simulink model "model"  (R2024b)
settings: Solver=ode45  StartTime=0.0  StopTime=1  FixedStep=0.0000001  MaxStep=1e-5  RelTol=1e-9  AbsTol=1e-9
InitFcn:
  | rs=0.435
  | Lls=0.754/(2*pi*60)
  | rr=0.816
  | Llr=0.754/(2*pi*60)
  | Lm=26.13/(2*pi*60)
  | J=0.0089; % 0.089
  | p=4;
  | Lss=Lls+Lm;
  | Lrr=Llr+Lm;
  | n= 1710; %rpm
  | Freq = 60;
  | 
  | Pbase= 3*746; % kw, 3hp
  | Vbase=220/sqrt(3)
  | Ibase= 8.2
  | Zbase = Vbase/Ibase
  | Lbase=Zbase/(2*pi*60)
  | Lm_pu = Lm/Lbase
  | Flx_pu = 1/Lm_pu
  | We_rated = 2*pi*Freq
  | Wm_rated = n/60*2*pi
  | T_rated = Pbase/Wm_rated
  | Flux_base = Vbase*sqrt(2)/We_rated
libraries: powerlib_extras x6, simulink_extras x1, spspowerguiLib x1
settings Model: Creator=Aditya  LastModifiedBy=tnt4
settings SolverCC: AutoScaleAbsTol=off  ZeroCrossAlgorithm=Adaptive  AlgebraicLoopSolver=TrustRegion
settings DataIOCC: SaveFormat=Array  SignalLoggingSaveFormat=ModelDataLogs  ReturnWorkspaceOutputs=off
settings OptimizationCC: BlockReduction=off  BooleanDataType=off  ExpressionDepthLimit=2147483647  InitFltsAndDblsToZero=on  LifeSpan=inf
settings DebuggingCC: SaveWithParameterizedLinksMsg=none  UnderspecifiedInitializationDetection=Classic  MergeDetectMultiDrivingBlocksExec=none  SignalResolutionControl=TryResolveAllWithWarning  MaxConsecutiveZCsMsg=none  MultiTaskDSMMsg=warning  MultiTaskCondExecSysMsg=none  FcnCallInpInsideContextMsg=warning  UnconnectedInputMsg=warning  UnconnectedOutputMsg=warning  UnconnectedLineMsg=warning  StateNameClashWarn=warning  SFUnexpectedBacktrackingDiag=warning  SFNoUnconditionalDefaultTransitionDiag=warning  SFExecutionAtInitializationDiag=none  ArithmeticOperatorsInVariantConditions=warning
settings HardwareCC: ProdBitPerPointer=32  ProdBitPerSizeT=32  ProdBitPerPtrDiffT=32  ProdLargestAtomicFloat=None  ProdIntDivRoundTo=Undefined  ProdEndianess=Unspecified  ProdWordSize=32  ProdHWDeviceType=32-bit Generic  TargetUnknown=on
settings ModelReferenceCC: EnableRefExpFcnMdlSchedulingChecks=on  PropagateSignalLabelsOutOfModel=off
settings SFSimCC: SimUseLocalCustomCode=off  CustomCodeUndefinedFunction=UseInterfaceOnly
settings RTWCC: TemplateMakefile=grt_unix.tmf  RTWUseLocalCustomCode=off  GPUComputeCapability=3.5
settings CodeAppCC: StateflowObjectComments=on
settings GRTTargetCC: TargetFcnLib=ansi_tfl_tmw.mat  TargetLangStandard=C89/C90 (ANSI)  CombineOutputUpdateFcns=off  GRTInterface=on
settings ConfigComp: CovMetricSettings=dw  CovSaveCumulativeToWorkspaceVar=on  CovSaveSingleToWorkspaceVar=on  CovExternalEMLEnable=off

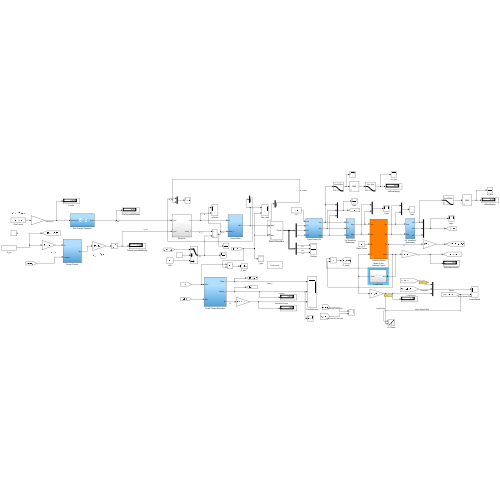
[thumbnail: Simulink's stored preview of the top-level diagram]
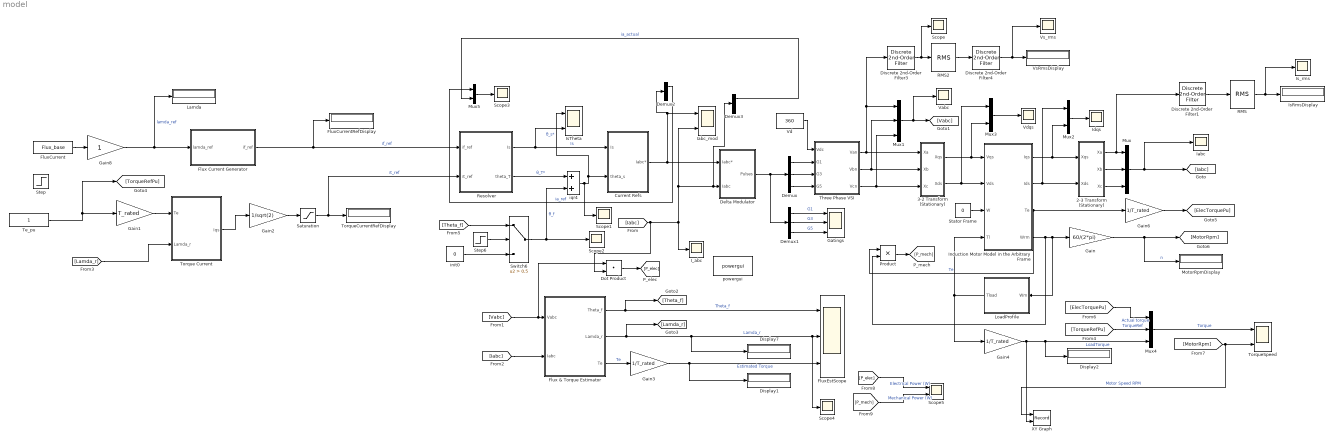
== system model ==
  2-3 Transform (Stationary) : Subsystem
  3-2 Transform (Stationary) : Subsystem
  Current Refs : Subsystem
  Delta Modulator : Subsystem  AncestorBlock=electricdrivelib/Fundamental Drive Blocks/Field-Oriented Controller/Detailed/Current Regulator  mask{h=Ibase*0.05}
      mask prompts: h "Modulator Band Width"
  Demux{,1..3} (4 alike) : Demux  Outputs=3
  Discrete 2nd-Order Filter1 : powerlib_extras/Discrete  Control Blocks/Discrete  2nd-Order Filter  FilterType=Lowpass  Fo=300  Zeta=0.5  Ts=50e-6  Initialize=off  Vac_Init=[0.8 -25 60]  Vdc_Init=-0.4  PlotResponse=off  param1=[1 500 1]
  Discrete 2nd-Order Filter3 : powerlib_extras/Discrete  Control Blocks/Discrete  2nd-Order Filter  FilterType=Lowpass  Fo=300  Zeta=0.5  Ts=50e-6  Initialize=off  Vac_Init=[0.8 -25 60]  Vdc_Init=-0.4  PlotResponse=off  param1=[1 500 1]
  Discrete 2nd-Order Filter4 : powerlib_extras/Discrete  Control Blocks/Discrete  2nd-Order Filter  FilterType=Lowpass  Fo=1  Zeta=0.5  Ts=50e-6  Initialize=off  Vac_Init=[0.8 -25 60]  Vdc_Init=-0.4  PlotResponse=off  param1=[1 500 1]
  Display1 : Display
  Display2 : Display
  Display7 : Display
  Dot Product : DotProduct  OutDataTypeStr=Inherit: Inherit via internal rule
  Flux & Torque Estimator : Subsystem
  Flux Current Generator : Subsystem
  FluxCurrent : Constant  Value=Flux_base
  FluxCurrentRefDisplay : Display
  FluxEstScope : Scope  NumInputPorts=3
  Gain : Gain  Gain=60/(2*pi)
  Gain1 : Gain  Gain=T_rated
  Gain2 : Gain  Gain=1/sqrt(2)
  Gain3 : Gain  Gain=1/T_rated
  Gain4 : Gain  Gain=1/T_rated
  Gain6 : Gain  Gain=1/T_rated
  Gain8 : Gain
  Gatings : Scope  NumInputPorts=3
  I_abc : Scope
  Iabc : Scope
  Iabc_mod : Scope  NumInputPorts=2
  Idqs : Scope
  Induction Motor Model in the Arbitrary Frame : Subsystem  mask{Rs=rs, Rr=rr, XLm=Lm, XLs=Lls, XLr=Llr, J=J}
  IsRmsDisplay : Display
  IsTheta : Scope  NumInputPorts=2
  Is_rms : Scope
  Lamda : Display
  LoadProfile : Subsystem
  MotorRpmDisplay : Display
  Mux : Mux  Inputs=3
  Mux1 : Mux  Inputs=3
  Mux2 : Mux  Inputs=2
  Mux3 : Mux  Inputs=2
  Mux4 : Mux  Inputs=3
  Mux5 : Mux  Inputs=2
  Product : Product
  RMS : powerlib_extras/Measurements/RMS  f1=60
  RMS2 : powerlib_extras/Measurements/RMS  f1=60
  Resolver : Subsystem
  Saturation : Saturate  UpperLimit=Ibase*1.5  LowerLimit=-Ibase*1.5
  Scope{,1..4} (5 alike) : Scope
  Scope5 : Scope  NumInputPorts=2
  Stator Frame : Constant  Value=0
  Step : Step  Time=0.5  Before=0.2  SampleTime=0
  Step6 : Step  Time=0.01  SampleTime=0
  Switch6 : Switch  Criteria=u2 > Threshold  Threshold=0.5  SaturateOnIntegerOverflow=off  InputSameDT=off
  Te_pu : Constant
  Three Phase VSI : Subsystem
  "Torque Current " : Subsystem
  TorqueCurrentRefDisplay : Display
  TorqueSpeed : Scope  NumInputPorts=2
  Vabc : Scope
  Vd : Constant  Value=360
  Vdqs : Scope
  VsRmsDisplay : Display
  Vs_rms : Scope
  XY Graph : Record  FileSettingsInternal="{\"entries\":[{\"content\":{\"excelSettings\":{\"content\":{},\"type\":\"Streamout.ExcelSettings\"}},\"type\":\"Streamout.FileSettingStorage\",\"uuid\":\"\"}],\"packageUris\":[\"http:\\/\\/schema.mathworks.com\\/mf0\\/streamout_blocks\\/R2020a\"],\"version\":\"1.0\"}"  Layout=[1 1]  SignalsInternal="{\"entries\":[{\"content\":{\"signals\":[{\"content\":{\"blockPath\":[],\"dimensions\":[1],\"domain\":\"\",\"lineColor\":\"#a2142f\",\"plots\":[ 1 ],\"port\":1,\"sid\":[\"\"],\"signalID\":1,\"signalName\":\"Motor Speed RPM\"},\"type\":\"RecordBlkView.Signal\",\"uuid\":\"\"},{\"content\":{\"blockPath\":[],\"dimensions\":[1],\"domain\":\"\",\"lineColor\":\"#139fff\",\"plots\":[ 1 ],\"port\":2,\"sid\":[\"\"],\"signalID\":2,\"signalName\":\"LoadTorque\"},\"type\":\"RecordBlkView.Signal\",\"uuid\":\"\"}]},\"type\":\"RecordBlkView.InputSignals\",\"uuid\":\"\"}],\"packageUris\":[\"http:\\/\\/schema.mathworks.com\\/mf0\\/streamout_blocks\\/R2020a\"],\"version\":\"1.0\"}"  VisualizationBindings="{\"xyplotplugin\":{\"info\":[{\"series\":[{\"bindingParametersList\":[{\"parameter\":\"X-Axis\",\"signalID\":1,\"signalName\":\"Motor Speed RPM\"},{\"parameter\":\"Y-Axis\",\"signalID\":2,\"signalName\":\"LoadTorque\"}],\"seriesID\":0}],\"subplotID\":1}]}}"  CompatibilityTag=XY
  init0 : Constant  Value=0
  iqr4 : Sum
  powergui : spspowerguiLib/powergui  Priority=1  SimulationMode=Continuous  SampleTime=50e-6  frequency=60  Iterations=50  frequencyindice=60  Pbase=100e6  ErrMax=1e-4  UnitsV=kV  UnitsW=MW  buscounter=0  FunctionMessages=off  echomessages=off  EnableUseOfTLC=off  CurrentSourceSwitches=off  DisableSnubberDevices=off  DisableRonSwitches=off  DisableVfSwitches=off  DisplayEquations=off  AutomaticDiscreteSolvers=off  SolverType=Tustin/Backward Euler (TBE)  Interpol=off  ExternalGateDelay=off  methode=off  Ts=100  x0status=blocks  SPID=on  SwTol=0  HookPort=off  NonlinearTolerance=1e-4  nMaxIteration=100  ContinueOnMaxIteration=off  RestoreLinks=warning  ResistiveCurrentMeasurement=off  Frange=[0:2:500]  Ylog=off  Xlog=on  ShowGrid=off  save=off  variable=ZData  structure=0  ZoomFFT=off  StartTime=0.0  cycles=1  DisplayStyle=1  fundamental=60  FreqAxis=off  MaxFrequency=1000  frequencyindicesteady=1  RmsSteady=1  display=off
  wires:
  3-2 Transform (Stationary)/1(Xqs) -> Mux3/2, Induction Motor Model in the Arbitrary Frame/1(Vqs)
  3-2 Transform (Stationary)/2(Xds) -> Mux3/1, Induction Motor Model in the Arbitrary Frame/2(Vds)
  Stator Frame/1 -> Induction Motor Model in the Arbitrary Frame/3(W)
  Induction Motor Model in the Arbitrary Frame/1(Iqs) -> Mux2/2, 2-3 Transform (Stationary)/1(Xqs)
  Induction Motor Model in the Arbitrary Frame/2(Ids) -> Mux2/1, 2-3 Transform (Stationary)/2(Xds)
  Induction Motor Model in the Arbitrary Frame/4(Wrm) -> Product/2, LoadProfile/1(Wm), Gain/1
  Gain/1 -> [MotorRpm], MotorRpmDisplay/1  "n"
  Vd/1 -> Three Phase VSI/1(Vdc)
  Demux/1 -> Three Phase VSI/2(G1)
  Demux/2 -> Three Phase VSI/3(G3)
  Demux/3 -> Three Phase VSI/4(G5)
  2-3 Transform (Stationary)/2(Xb) -> Mux/2
  2-3 Transform (Stationary)/3(Xc) -> Mux/3
  2-3 Transform (Stationary)/1(Xa) -> Discrete 2nd-Order Filter1/1, Mux/1
  Three Phase VSI/1(Van) -> Discrete 2nd-Order Filter3/1, Mux1/1, 3-2 Transform (Stationary)/1(Xa)
  Three Phase VSI/2(Vbn) -> Mux1/2, 3-2 Transform (Stationary)/2(Xb)
  Three Phase VSI/3(Vcn) -> Mux1/3, 3-2 Transform (Stationary)/3(Xc)
  Mux1/1 -> Vabc/1, [Vabc]
  [Iabc] -> Dot Product/2, I_abc/1, Iabc_mod/2, Demux3/1, Delta Modulator/2(Iabc)
  Current Refs/1(Iabc*) -> Demux2/1, Iabc_mod/1, Delta Modulator/1(Iabc*)
  [Vabc] -> Dot Product/1, Flux & Torque Estimator/1(Vabc)
  [Iabc] -> Flux & Torque Estimator/2(Iabc)
  Flux & Torque Estimator/1(Theta_f) -> [Theta_f], FluxEstScope/1  "Theta_f"
  Flux & Torque Estimator/3(Te) -> Gain3/1  "Te"
  Induction Motor Model in the Arbitrary Frame/3(Te) -> Product/1, Gain6/1  "Te"
  Mux/1 -> [Iabc], Iabc/1
  Flux & Torque Estimator/2(Lamda_r) -> [Lamda_r], Display7/1, Scope4/1, FluxEstScope/2  "Lamda_r"
  FluxCurrent/1 -> Gain8/1
  iqr4/1 -> Scope1/1, IsTheta/1, Current Refs/2(theta_s)  "θ_s*"
  Delta Modulator/1(Pulses) -> Demux1/1, Demux/1
  Demux1/3 -> Gatings/3  "G5"
  Demux1/2 -> Gatings/2  "G3"
  Demux1/1 -> Gatings/1  "G1"
  Mux2/1 -> Idqs/1
  Mux3/1 -> Vdqs/1
  LoadProfile/1(Tload) -> Gain4/1, Induction Motor Model in the Arbitrary Frame/4(Tl)
  Gain3/1 -> Display1/1, FluxEstScope/3  "Estimated Torque"
  Discrete 2nd-Order Filter1/1 -> RMS/1
  RMS/1 -> Is_rms/1, IsRmsDisplay/1
  "Torque Current "/1(Iqs) -> Gain2/1
  Gain1/1 -> "Torque Current "/1(Te)
  Gain2/1 -> Saturation/1
  [Lamda_r] -> "Torque Current "/2(Lamda_r)
  Saturation/1 -> Resolver/2(it_ref), TorqueCurrentRefDisplay/1  "it_ref"
  RMS2/1 -> Discrete 2nd-Order Filter4/1
  Discrete 2nd-Order Filter3/1 -> Scope/1, RMS2/1
  Discrete 2nd-Order Filter4/1 -> Vs_rms/1, VsRmsDisplay/1
  Gain4/1 -> XY Graph/2, Display2/1, Mux4/3  "LoadTorque"
  [TorqueRefPu] -> Mux4/2  "TorqueRef"
  Gain6/1 -> [ElecTorquePu]
  [ElecTorquePu] -> Mux4/1  "Actual torque"
  Mux4/1 -> TorqueSpeed/1  "Torque"
  [MotorRpm] -> XY Graph/1, TorqueSpeed/2  "Motor Speed RPM"
  Gain8/1 -> Lamda/1, Flux Current Generator/1(lamda_ref)  "lamda_ref"
  [Theta_f] -> Switch6/1
  Step6/1 -> Switch6/2
  init0/1 -> Switch6/3
  Resolver/1(Is) -> IsTheta/2, Current Refs/1(Is)  "Is"
  Resolver/2(theta_T) -> iqr4/1  "θ_T*"
  Flux Current Generator/1(if_ref) -> FluxCurrentRefDisplay/1, Resolver/1(if_ref)  "if_ref"
  Switch6/1 -> iqr4/2, Scope2/1  "θ_f"
  Mux5/1 -> Scope3/1
  Demux2/1 -> Mux5/1  "ia_ref"
  Demux3/1 -> Mux5/2  "ia_actual"
  Te_pu/1 -> Gain1/1, [TorqueRefPu]
  Dot Product/1 -> [P_elec]
  Product/1 -> [P_mech]
  [P_elec] -> Scope5/1  "Electrical Power (W)"
  [P_mech] -> Scope5/2  "Mechanical Power (W)"

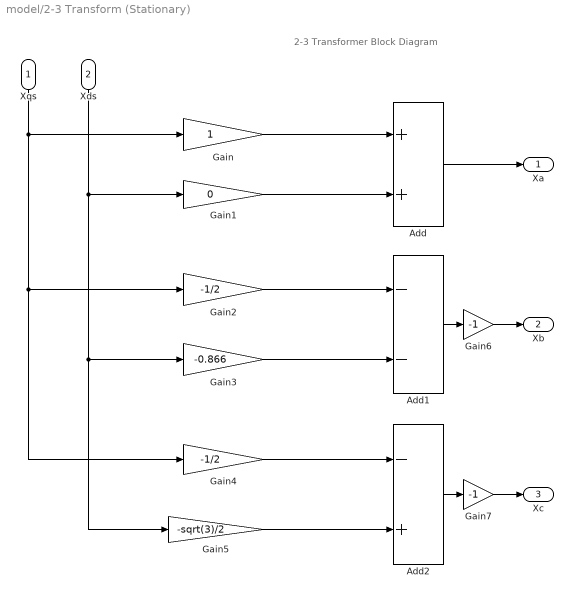
== system model/2-3 Transform (Stationary) ==
  note: 2-3 Transformer Block Diagram
  Xqs : Inport
  Xds : Inport  Port=2
  Add : Sum
  Add1 : Sum  Inputs=--
  Add2 : Sum  Inputs=-+
  Gain : Gain
  Gain1 : Gain  Gain=0
  Gain2 : Gain  Gain=-1/2
  Gain3 : Gain  Gain=-0.866
  Gain4 : Gain  Gain=-1/2
  Gain5 : Gain  Gain=-sqrt(3)/2
  Gain6 : Gain  Gain=-1
  Gain7 : Gain  Gain=-1
  Xa : Outport  VectorParamsAs1DForOutWhenUnconnected=off
  Xb : Outport  Port=2  VectorParamsAs1DForOutWhenUnconnected=off
  Xc : Outport  Port=3  VectorParamsAs1DForOutWhenUnconnected=off
  wires:
  Add2/1 -> Gain7/1
  Gain/1 -> Add/1
  Gain3/1 -> Add1/2
  Gain5/1 -> Add2/2
  Gain1/1 -> Add/2
  Gain7/1 -> Xc/1
  Xds/1 -> Gain1/1, Gain3/1, Gain5/1
  Add1/1 -> Gain6/1
  Gain2/1 -> Add1/1
  Xqs/1 -> Gain/1, Gain2/1, Gain4/1
  Gain6/1 -> Xb/1
  Gain4/1 -> Add2/1
  Add/1 -> Xa/1

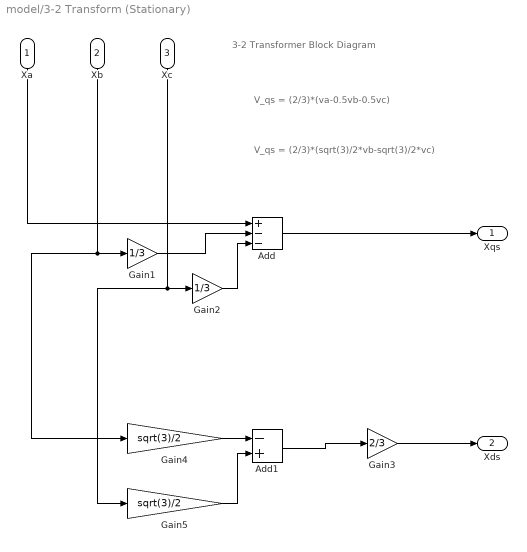
== system model/3-2 Transform (Stationary) ==
  note: 3-2 Transformer Block Diagram
  note: V_qs = (2/3)*(sqrt(3)/2*vb-sqrt(3)/2*vc)
  note: V_qs = (2/3)*(va-0.5vb-0.5vc)
  Xa : Inport
  Xb : Inport  Port=2
  Xc : Inport  Port=3
  Add : Sum  Inputs=+--
  Add1 : Sum  Inputs=-+
  Gain1 : Gain  Gain=1/3
  Gain2 : Gain  Gain=1/3
  Gain3 : Gain  Gain=2/3
  Gain4 : Gain  Gain=sqrt(3)/2
  Gain5 : Gain  Gain=sqrt(3)/2
  Xqs : Outport  VectorParamsAs1DForOutWhenUnconnected=off
  Xds : Outport  Port=2  VectorParamsAs1DForOutWhenUnconnected=off
  wires:
  Gain5/1 -> Add1/2
  Add/1 -> Xqs/1
  Add1/1 -> Gain3/1
  Gain1/1 -> Add/2
  Gain2/1 -> Add/3
  Xa/1 -> Add/1
  Xc/1 -> Gain5/1, Gain2/1
  Xb/1 -> Gain4/1, Gain1/1
  Gain4/1 -> Add1/1
  Gain3/1 -> Xds/1

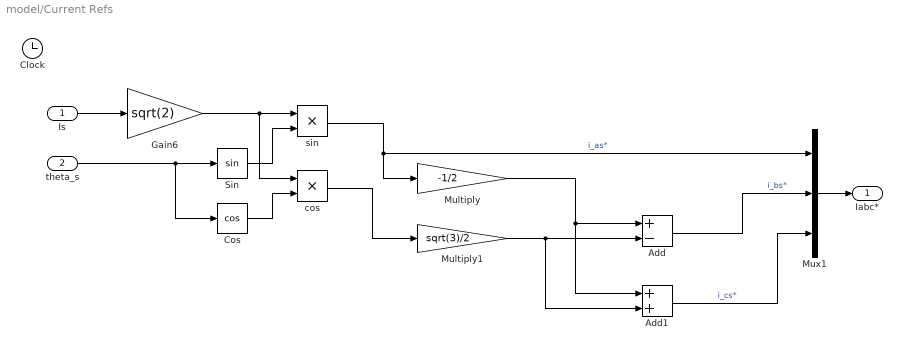
== system model/Current Refs ==
  Is : Inport
  theta_s : Inport  Port=2
  Add : Sum  Inputs=+-
  Add1 : Sum
  Clock : Clock
  Cos : Trigonometry  Operator=cos
  Gain6 : Gain  Gain=sqrt(2)
  Multiply : Gain  Gain=-1/2
  Multiply1 : Gain  Gain=sqrt(3)/2
  Mux1 : Mux  Inputs=3
  Sin : Trigonometry
  cos : Product
  sin : Product
  Iabc* : Outport  VectorParamsAs1DForOutWhenUnconnected=off
  wires:
  Mux1/1 -> Iabc*/1
  Is/1 -> Gain6/1
  cos/1 -> Multiply1/1
  sin/1 -> Mux1/1, Multiply/1  "i_as*"
  Add/1 -> Mux1/2  "i_bs*"
  Multiply1/1 -> Add1/2, Add/2
  Multiply/1 -> Add1/1, Add/1
  Add1/1 -> Mux1/3  "i_cs*"
  Sin/1 -> sin/2
  Cos/1 -> cos/2
  Gain6/1 -> cos/1, sin/1
  theta_s/1 -> Cos/1, Sin/1

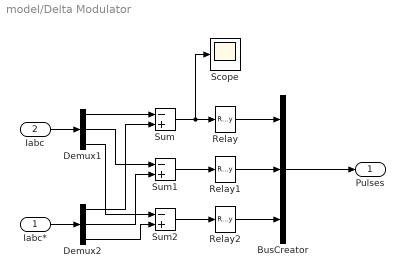
== system model/Delta Modulator ==
  Iabc* : Inport
  Iabc : Inport  Port=2
  BusCreator : BusCreator  Inputs=3
  Demux1 : Demux  Outputs=3
      settings: DisplayOption=none
  Demux2 : Demux  Outputs=3
      settings: DisplayOption=none
  Relay : Relay  OnSwitchValue=1/2  OffSwitchValue=-1/2
  Relay1 : Relay  OnSwitchValue=1/2  OffSwitchValue=-1/2
  Relay2 : Relay  OnSwitchValue=1/2  OffSwitchValue=-1/2
  Scope : Scope
  Sum : Sum  Inputs=-+  InputSameDT=on  SaturateOnIntegerOverflow=on  OutDataTypeStr=Inherit: Same as first input
  Sum1 : Sum  Inputs=-+  InputSameDT=on  SaturateOnIntegerOverflow=on  OutDataTypeStr=Inherit: Same as first input
  Sum2 : Sum  Inputs=-+  InputSameDT=on  SaturateOnIntegerOverflow=on  OutDataTypeStr=Inherit: Same as first input
  Pulses : Outport  InitialOutput=0  VectorParamsAs1DForOutWhenUnconnected=off
  wires:
  Sum/1 -> Scope/1, Relay/1
  Sum1/1 -> Relay1/1
  Demux1/1 -> Sum/1
  Demux1/2 -> Sum1/1
  BusCreator/1 -> Pulses/1
  Iabc/1 -> Demux1/1
  Sum2/1 -> Relay2/1
  Demux1/3 -> Sum2/1
  Demux2/3 -> Sum2/2
  Demux2/2 -> Sum1/2
  Demux2/1 -> Sum/2
  Iabc*/1 -> Demux2/1
  Relay/1 -> BusCreator/1
  Relay1/1 -> BusCreator/2
  Relay2/1 -> BusCreator/3

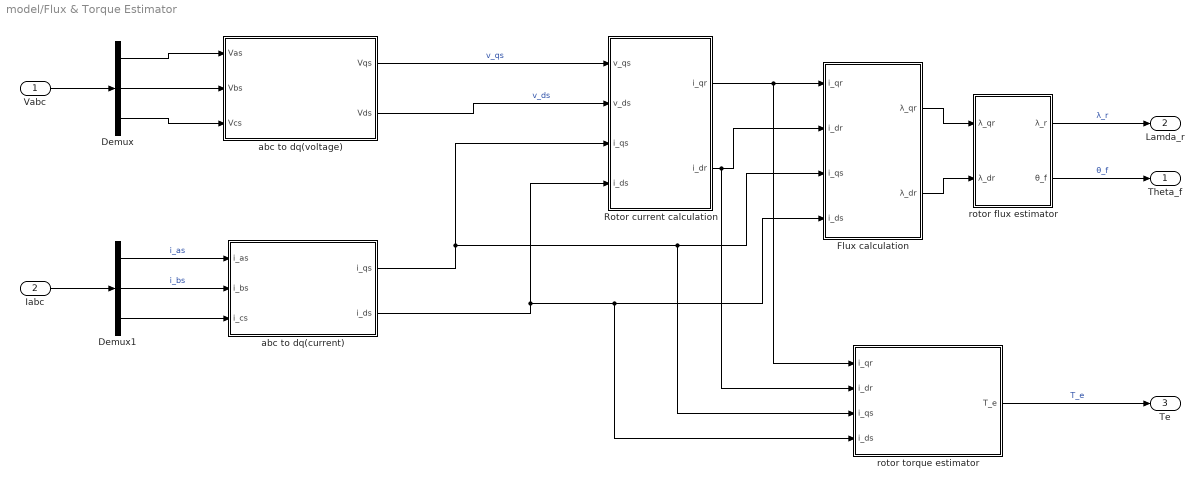
== system model/Flux & Torque Estimator ==
  Vabc : Inport
  Iabc : Inport  Port=2
  Demux : Demux  Outputs=3
  Demux1 : Demux  Outputs=3
  Flux calculation : Subsystem
  Rotor current calculation : Subsystem
  abc to dq(current) : Subsystem
  abc to dq(voltage) : Subsystem
  rotor flux estimator : Subsystem
  rotor torque estimator : Subsystem
  Theta_f : Outport  OutDataTypeStr=double  VectorParamsAs1DForOutWhenUnconnected=off
  Lamda_r : Outport  Port=2  VectorParamsAs1DForOutWhenUnconnected=off
  Te : Outport  Port=3  VectorParamsAs1DForOutWhenUnconnected=off
  wires:
  Vabc/1 -> Demux/1
  Iabc/1 -> Demux1/1
  abc to dq(current)/2(i_ds) -> rotor torque estimator/4(i_ds), Flux calculation/4(i_ds), Rotor current calculation/4(i_ds)
  abc to dq(voltage)/1(Vqs) -> Rotor current calculation/1(v_qs)  "v_qs"
  Rotor current calculation/1(i_qr) -> rotor torque estimator/1(i_qr), Flux calculation/1(i_qr)
  Flux calculation/2(λ_dr) -> rotor flux estimator/2(λ_dr)
  Demux/2 -> abc to dq(voltage)/2(Vbs)
  rotor flux estimator/2(θ_f) -> Theta_f/1  "θ_f"
  Rotor current calculation/2(i_dr) -> rotor torque estimator/2(i_dr), Flux calculation/2(i_dr)
  rotor torque estimator/1(T_e) -> Te/1  "T_e"
  rotor flux estimator/1(λ_r) -> Lamda_r/1  "λ_r"
  abc to dq(current)/1(i_qs) -> Rotor current calculation/3(i_qs), rotor torque estimator/3(i_qs), Flux calculation/3(i_qs)
  abc to dq(voltage)/2(Vds) -> Rotor current calculation/2(v_ds)  "v_ds"
  Flux calculation/1(λ_qr) -> rotor flux estimator/1(λ_qr)
  Demux1/1 -> abc to dq(current)/1(i_as)  "i_as"
  Demux/1 -> abc to dq(voltage)/1(Vas)
  Demux/3 -> abc to dq(voltage)/3(Vcs)
  Demux1/2 -> abc to dq(current)/2(i_bs)  "i_bs"
  Demux1/3 -> abc to dq(current)/3(i_cs)

== system model/Flux Current Generator ==
  lamda_ref : Inport
  Gain7 : Gain  Gain=1/Lm
  Gain9 : Gain  Gain=1/sqrt(2)
  if_ref : Outport
  wires:
  Gain7/1 -> Gain9/1
  Gain9/1 -> if_ref/1  "if_ref"
  lamda_ref/1 -> Gain7/1

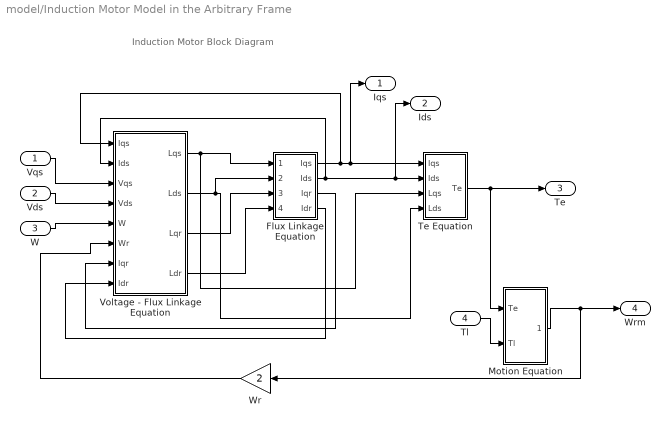
== system model/Induction Motor Model in the Arbitrary Frame ==
  note: Induction Motor Block Diagram
  Vqs : Inport
  Vds : Inport  Port=2
  W : Inport  Port=3
  Tl : Inport  Port=4
  Flux Linkage Equation : Subsystem
  Motion Equation : Subsystem
  Te Equation : Subsystem
  Voltage - Flux Linkage Equation : Subsystem
  Wr : Gain  Gain=2
  Iqs : Outport  VectorParamsAs1DForOutWhenUnconnected=off
  Ids : Outport  Port=2  VectorParamsAs1DForOutWhenUnconnected=off
  Te : Outport  Port=3  VectorParamsAs1DForOutWhenUnconnected=off
  Wrm : Outport  Port=4  VectorParamsAs1DForOutWhenUnconnected=off
  wires:
  Flux Linkage Equation/1(Iqs) -> Voltage - Flux Linkage Equation/1(Iqs), Te Equation/1(Iqs), Iqs/1
  Flux Linkage Equation/2(Ids) -> Voltage - Flux Linkage Equation/2(Ids), Te Equation/2(Ids), Ids/1
  Te Equation/1(Te) -> Motion Equation/1(Te), Te/1
  Motion Equation/1(Wrm) -> Wr/1, Wrm/1
  Wr/1 -> Voltage - Flux Linkage Equation/6(Wr)
  Flux Linkage Equation/3(Iqr) -> Voltage - Flux Linkage Equation/7(Iqr)
  Flux Linkage Equation/4(Idr) -> Voltage - Flux Linkage Equation/8(Idr)
  Vqs/1 -> Voltage - Flux Linkage Equation/3(Vqs)
  Vds/1 -> Voltage - Flux Linkage Equation/4(Vds)
  W/1 -> Voltage - Flux Linkage Equation/5(W)
  Tl/1 -> Motion Equation/2(Tl)
  Voltage - Flux Linkage Equation/1(Lqs) -> Flux Linkage Equation/1(Lqs), Te Equation/3(Lqs)
  Voltage - Flux Linkage Equation/2(Lds) -> Flux Linkage Equation/2(Lds), Te Equation/4(Lds)
  Voltage - Flux Linkage Equation/3(Lqr) -> Flux Linkage Equation/3(Lqr)
  Voltage - Flux Linkage Equation/4(Ldr) -> Flux Linkage Equation/4(Ldr)

== system model/LoadProfile ==
  Wm : Inport
  Add : Sum
  FanTypeTrqGain : Constant  Value=T_rated/(Wm_rated^2)
  Multiply1 : Product  Inputs=3
  Step : Step  Time=0.5  After=0  SampleTime=0
  Tload : Outport  VectorParamsAs1DForOutWhenUnconnected=off
  wires:
  Wm/1 -> Multiply1/2, Multiply1/1
  FanTypeTrqGain/1 -> Multiply1/3
  Multiply1/1 -> Add/1
  Step/1 -> Add/2
  Add/1 -> Tload/1

== system model/Resolver ==
  if_ref : Inport
  it_ref : Inport  Port=2
  Cartesian to Polar : simulink_extras/Transformations/Cartesian to Polar
  Is : Outport
  theta_T : Outport  Port=2
  wires:
  Cartesian to Polar/2 -> theta_T/1  "theta_T"
  Cartesian to Polar/1 -> Is/1  "Is"
  it_ref/1 -> Cartesian to Polar/2
  if_ref/1 -> Cartesian to Polar/1

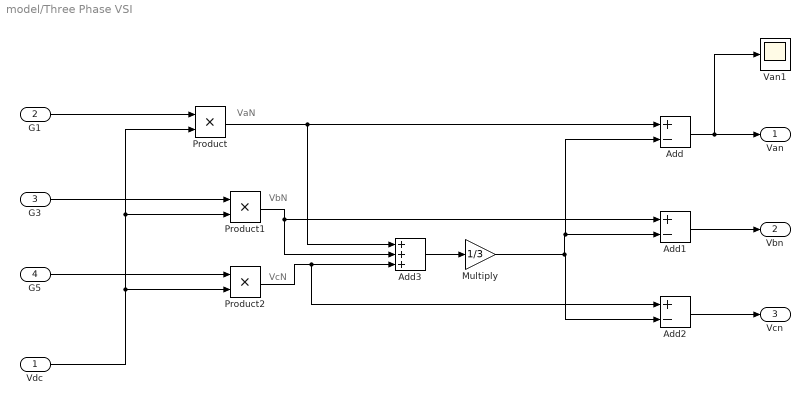
== system model/Three Phase VSI ==
  note: VaN
  note: VbN
  note: VcN
  Vdc : Inport
  G1 : Inport  Port=2
  G3 : Inport  Port=3
  G5 : Inport  Port=4
  Add : Sum  Inputs=+-
  Add1 : Sum  Inputs=+-
  Add2 : Sum  Inputs=+-
  Add3 : Sum  Inputs=+++
  Multiply : Gain  Gain=1/3
  Product : Product
  Product1 : Product
  Product2 : Product
  Van1 : Scope
  Van : Outport  OutDataTypeStr=double  VectorParamsAs1DForOutWhenUnconnected=off
  Vbn : Outport  Port=2  VectorParamsAs1DForOutWhenUnconnected=off
  Vcn : Outport  Port=3  VectorParamsAs1DForOutWhenUnconnected=off
  wires:
  Multiply/1 -> Add/2, Add1/2, Add2/2
  Product2/1 -> Add2/1, Add3/3
  Vdc/1 -> Product2/2, Product1/2, Product/2
  G5/1 -> Product2/1
  Product/1 -> Add3/1, Add/1
  Product1/1 -> Add1/1, Add3/2
  Add3/1 -> Multiply/1
  Add1/1 -> Vbn/1
  Add/1 -> Van1/1, Van/1
  G3/1 -> Product1/1
  Add2/1 -> Vcn/1
  G1/1 -> Product/1

== system model/Torque Current  ==
  Te : Inport
  Lamda_r : Inport  Port=2
  Constant : Constant  Value=0.001
  Constant1 : Constant  Value=(3/2)*(p/2)*(Lm/Lrr)
  Discrete 2nd-Order Filter2 : powerlib_extras/Discrete  Control Blocks/Discrete  2nd-Order Filter  FilterType=Lowpass  Fo=60  Zeta=0.5  Ts=50e-6  Initialize=off  Vac_Init=[0.8 -25 60]  Vdc_Init=-0.4  PlotResponse=off  param1=[1 500 1]
  Divide : Product  Inputs=*/
  Product : Product
  prevent division by zero / huge spikes : MinMax  Function=max  Inputs=2
  Iqs : Outport  VectorParamsAs1DForOutWhenUnconnected=off
  wires:
  Lamda_r/1 -> Discrete 2nd-Order Filter2/1
  Constant/1 -> prevent division by zero / huge spikes/2
  Discrete 2nd-Order Filter2/1 -> prevent division by zero / huge spikes/1
  Constant1/1 -> Product/2
  Product/1 -> Divide/2
  prevent division by zero / huge spikes/1 -> Product/1
  Te/1 -> Divide/1
  Divide/1 -> Iqs/1  "i_qs*"

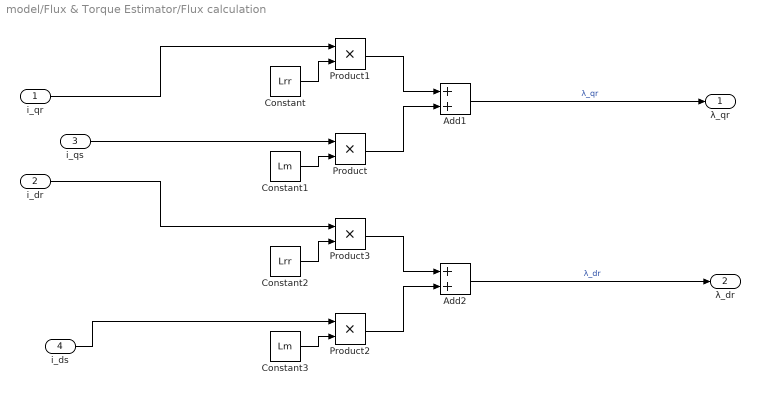
== system model/Flux & Torque Estimator/Flux calculation ==
  i_qr : Inport
  i_dr : Inport  Port=2
  i_qs : Inport  Port=3
  i_ds : Inport  Port=4
  Add1 : Sum
  Add2 : Sum
  Constant : Constant  Value=Lrr
  Constant1 : Constant  Value=Lm
  Constant2 : Constant  Value=Lrr
  Constant3 : Constant  Value=Lm
  Product{,1..3} (4 alike) : Product
  λ_qr : Outport
  λ_dr : Outport  Port=2
  wires:
  Constant/1 -> Product1/2
  Product/1 -> Add1/2
  i_qr/1 -> Product1/1
  Product2/1 -> Add2/2
  Constant3/1 -> Product2/2
  Product3/1 -> Add2/1
  i_dr/1 -> Product3/1
  Product1/1 -> Add1/1
  Constant2/1 -> Product3/2
  Constant1/1 -> Product/2
  i_qs/1 -> Product/1
  Add1/1 -> λ_qr/1  "λ_qr"
  Add2/1 -> λ_dr/1  "λ_dr"
  i_ds/1 -> Product2/1

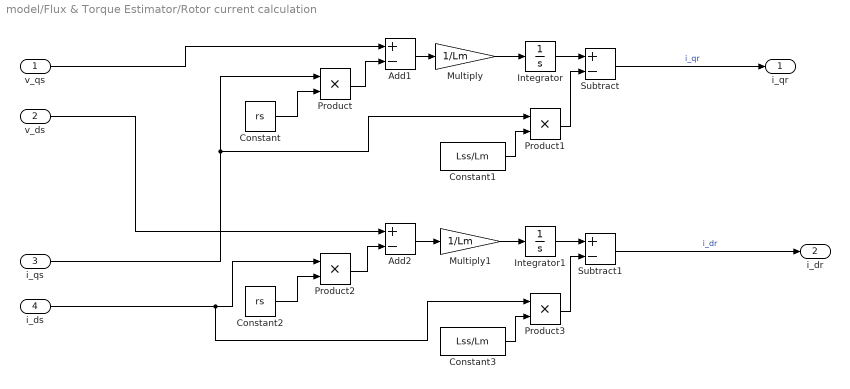
== system model/Flux & Torque Estimator/Rotor current calculation ==
  v_qs : Inport
  v_ds : Inport  Port=2
  i_qs : Inport  Port=3
  i_ds : Inport  Port=4
  Add1 : Sum  Inputs=+-
  Add2 : Sum  Inputs=+-
  Constant : Constant  Value=rs
  Constant1 : Constant  Value=Lss/Lm
  Constant2 : Constant  Value=rs
  Constant3 : Constant  Value=Lss/Lm
  Integrator : Integrator
  Integrator1 : Integrator
  Multiply : Gain  Gain=1/Lm
  Multiply1 : Gain  Gain=1/Lm
  Product{,1..3} (4 alike) : Product
  Subtract : Sum  Inputs=+-
  Subtract1 : Sum  Inputs=+-
  i_qr : Outport
  i_dr : Outport  Port=2
  wires:
  Integrator/1 -> Subtract/1
  i_qs/1 -> Product1/1, Product/1
  Constant2/1 -> Product2/2
  Product1/1 -> Subtract/2
  Constant3/1 -> Product3/2
  Product3/1 -> Subtract1/2
  Integrator1/1 -> Subtract1/1
  Product/1 -> Add1/2
  Constant1/1 -> Product1/2
  Product2/1 -> Add2/2
  i_ds/1 -> Product3/1, Product2/1
  Constant/1 -> Product/2
  v_ds/1 -> Add2/1
  Subtract1/1 -> i_dr/1  "i_dr"
  Subtract/1 -> i_qr/1  "i_qr"
  v_qs/1 -> Add1/1
  Add1/1 -> Multiply/1
  Multiply/1 -> Integrator/1
  Add2/1 -> Multiply1/1
  Multiply1/1 -> Integrator1/1

== system model/Flux & Torque Estimator/abc to dq(current) ==
  i_as : Inport
  i_bs : Inport  Port=2
  i_cs : Inport  Port=3
  Gain : Gain  Gain=(2/3)*(-1/2)
  Gain1 : Gain  Gain=(2/3)*(-1/2)
  Gain2 : Gain  Gain=(2/3)
  Gain4 : Gain  Gain=(2/3)*(-sqrt(3)/2)
  Gain5 : Gain  Gain=(2/3)*(sqrt(3)/2)
  Sum : Sum  Inputs=|+++
  Sum1 : Sum  Inputs=|++
  i_qs : Outport  InitialOutput=0  VectorParamsAs1DForOutWhenUnconnected=off
  i_ds : Outport  Port=2  InitialOutput=0  VectorParamsAs1DForOutWhenUnconnected=off
  wires:
  i_as/1 -> Gain2/1
  i_bs/1 -> Gain4/1, Gain/1
  Gain5/1 -> Sum1/1
  Gain4/1 -> Sum1/2
  Gain/1 -> Sum/2
  Sum1/1 -> i_ds/1
  Gain2/1 -> Sum/3
  i_cs/1 -> Gain5/1, Gain1/1
  Gain1/1 -> Sum/1
  Sum/1 -> i_qs/1

== system model/Flux & Torque Estimator/abc to dq(voltage) ==
  Vas : Inport
  Vbs : Inport  Port=2
  Vcs : Inport  Port=3
  Gain : Gain  Gain=(2/3)*(-1/2)
  Gain1 : Gain  Gain=(2/3)*(-1/2)
  Gain2 : Gain  Gain=(2/3)
  Gain4 : Gain  Gain=(2/3)*(-sqrt(3)/2)
  Gain5 : Gain  Gain=(2/3)*(sqrt(3)/2)
  Sum : Sum  Inputs=|+++
  Sum1 : Sum  Inputs=|++
  Vqs : Outport  InitialOutput=0  VectorParamsAs1DForOutWhenUnconnected=off
  Vds : Outport  Port=2  InitialOutput=0  VectorParamsAs1DForOutWhenUnconnected=off
  wires:
  Vas/1 -> Gain2/1
  Gain4/1 -> Sum1/2
  Gain2/1 -> Sum/3
  Vcs/1 -> Gain5/1, Gain1/1
  Gain5/1 -> Sum1/1
  Vbs/1 -> Gain4/1, Gain/1
  Gain1/1 -> Sum/1
  Sum1/1 -> Vds/1
  Gain/1 -> Sum/2
  Sum/1 -> Vqs/1

== system model/Flux & Torque Estimator/rotor flux estimator ==
  λ_qr : Inport
  λ_dr : Inport  Port=2
  Add1 : Sum
  Atan2 : Trigonometry  Operator=atan2
  Square : Math  Operator=square
  Square Root : Sqrt
  Square1 : Math  Operator=square
  λ_r : Outport
  θ_f : Outport  Port=2
  wires:
  Square/1 -> Add1/1
  λ_qr/1 -> Atan2/1, Square/1
  Square1/1 -> Add1/2
  Add1/1 -> Square Root/1
  Square Root/1 -> λ_r/1  "λ_r"
  λ_dr/1 -> Atan2/2, Square1/1
  Atan2/1 -> θ_f/1  "θ_f"

== system model/Flux & Torque Estimator/rotor torque estimator ==
  i_qr : Inport
  i_dr : Inport  Port=2
  i_qs : Inport  Port=3
  i_ds : Inport  Port=4
  Add1 : Sum  Inputs=+-
  Constant : Constant  Value=(3/2)*(p/2)*Lm
  Product : Product
  Product1 : Product
  Product2 : Product
  T_e : Outport
  wires:
  Product2/1 -> Add1/2
  i_ds/1 -> Product2/1
  Constant/1 -> Product/2
  Product1/1 -> Add1/1
  Add1/1 -> Product/1
  i_qs/1 -> Product1/1
  i_dr/1 -> Product1/2
  i_qr/1 -> Product2/2
  Product/1 -> T_e/1  "T_e"

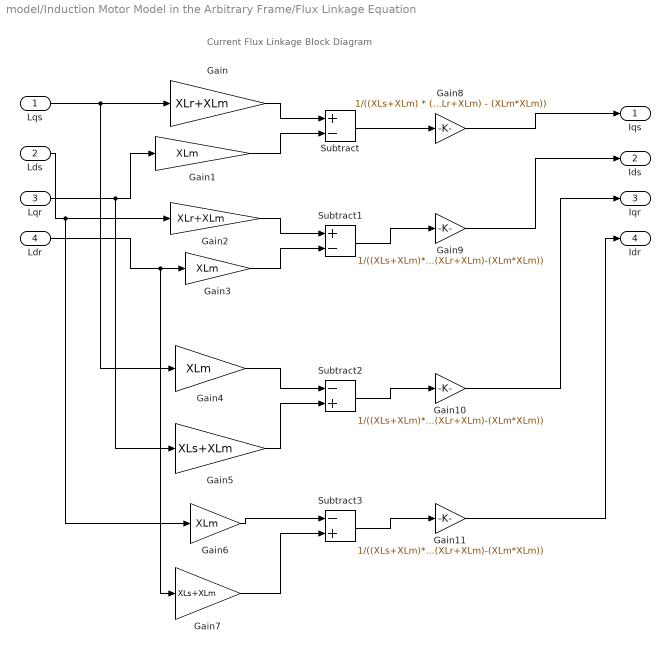
== system model/Induction Motor Model in the Arbitrary Frame/Flux Linkage Equation ==
  note: Current Flux Linkage Block Diagram
  Lqs : Inport
  Lds : Inport  Port=2
  Lqr : Inport  Port=3
  Ldr : Inport  Port=4
  Gain : Gain  Gain=XLr+XLm
  Gain{1,3..4,6} (4 alike) : Gain  Gain=XLm
  Gain10 : Gain  Gain=1/((XLs+XLm)*(XLr+XLm)-(XLm*XLm))
  Gain11 : Gain  Gain=1/((XLs+XLm)*(XLr+XLm)-(XLm*XLm))
  Gain2 : Gain  Gain=XLr+XLm
  Gain5 : Gain  Gain=XLs+XLm
  Gain7 : Gain  Gain=XLs+XLm
  Gain8 : Gain  Gain=1/((XLs+XLm) * (XLr+XLm) - (XLm*XLm))
  Gain9 : Gain  Gain=1/((XLs+XLm)*(XLr+XLm)-(XLm*XLm))
  Subtract : Sum  Inputs=+-
  Subtract1 : Sum  Inputs=+-
  Subtract2 : Sum  Inputs=-+
  Subtract3 : Sum  Inputs=-+
  Iqs : Outport  VectorParamsAs1DForOutWhenUnconnected=off
  Ids : Outport  Port=2  VectorParamsAs1DForOutWhenUnconnected=off
  Iqr : Outport  Port=3  VectorParamsAs1DForOutWhenUnconnected=off
  Idr : Outport  Port=4  VectorParamsAs1DForOutWhenUnconnected=off
  wires:
  Gain/1 -> Subtract/1
  Gain1/1 -> Subtract/2
  Lqs/1 -> Gain/1, Gain4/1
  Lqr/1 -> Gain1/1, Gain5/1
  Lds/1 -> Gain2/1, Gain6/1
  Ldr/1 -> Gain3/1, Gain7/1
  Gain2/1 -> Subtract1/1
  Gain3/1 -> Subtract1/2
  Gain4/1 -> Subtract2/1
  Gain5/1 -> Subtract2/2
  Gain6/1 -> Subtract3/1
  Gain7/1 -> Subtract3/2
  Subtract/1 -> Gain8/1
  Subtract1/1 -> Gain9/1
  Subtract2/1 -> Gain10/1
  Subtract3/1 -> Gain11/1
  Gain8/1 -> Iqs/1
  Gain9/1 -> Ids/1
  Gain10/1 -> Iqr/1
  Gain11/1 -> Idr/1

== system model/Induction Motor Model in the Arbitrary Frame/Motion Equation ==
  note: Motion Block Diagram
  Te : Inport
  Tl : Inport  Port=2
  Add : Sum  Inputs=+-
  Gain : Gain  Gain=1/J
  Integrator : Integrator
  Wrm : Outport  VectorParamsAs1DForOutWhenUnconnected=off
  wires:
  Te/1 -> Add/1
  Tl/1 -> Add/2
  Add/1 -> Gain/1
  Gain/1 -> Integrator/1
  Integrator/1 -> Wrm/1

== system model/Induction Motor Model in the Arbitrary Frame/Te Equation ==
  note: Te Block Diagram
  Iqs : Inport
  Ids : Inport  Port=2
  Lqs : Inport  Port=3
  Lds : Inport  Port=4
  Gain : Gain  Gain=3
  Product : Product  RndMeth=Zero
  Product1 : Product  RndMeth=Zero
  Subtract : Sum  Inputs=+-
  Te : Outport  VectorParamsAs1DForOutWhenUnconnected=off
  wires:
  Subtract/1 -> Gain/1
  Gain/1 -> Te/1
  Product/1 -> Subtract/1
  Product1/1 -> Subtract/2
  Lds/1 -> Product/1
  Iqs/1 -> Product/2
  Lqs/1 -> Product1/1
  Ids/1 -> Product1/2

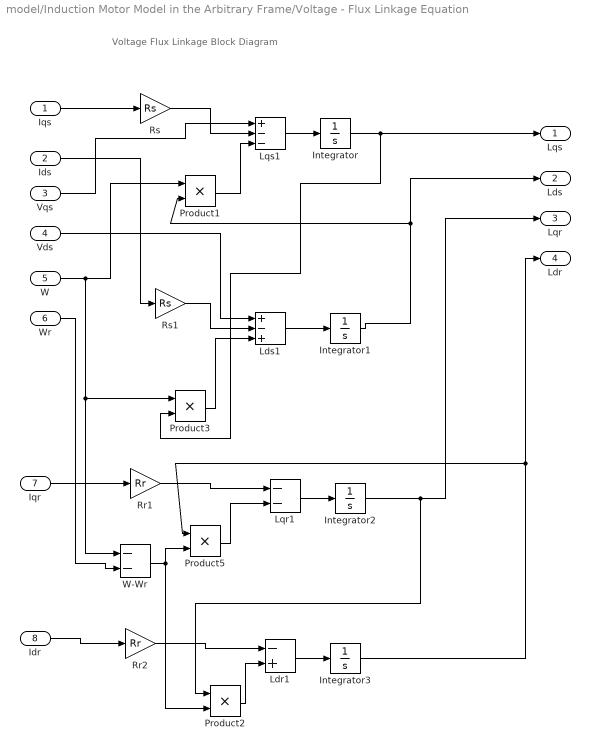
== system model/Induction Motor Model in the Arbitrary Frame/Voltage - Flux Linkage Equation ==
  note: Voltage Flux Linkage Block Diagram
  Iqs : Inport
  Ids : Inport  Port=2
  Vqs : Inport  Port=3
  Vds : Inport  Port=4
  W : Inport  Port=5
  Wr : Inport  Port=6
  Iqr : Inport  Port=7
  Idr : Inport  Port=8
  Integrator{,1..3} (4 alike) : Integrator
  Ldr1 : Sum  Inputs=-+
  Lds1 : Sum  Inputs=+-+
  Lqr1 : Sum  Inputs=--
  Lqs1 : Sum  Inputs=+--
  Product{1..3,5} (4 alike) : Product  RndMeth=Zero
  Rr1 : Gain  Gain=Rr
  Rr2 : Gain  Gain=Rr
  Rs : Gain  Gain=Rs
  Rs1 : Gain  Gain=Rs
  W-Wr : Sum  Inputs=--
  Lqs : Outport  VectorParamsAs1DForOutWhenUnconnected=off
  Lds : Outport  Port=2  VectorParamsAs1DForOutWhenUnconnected=off
  Lqr : Outport  Port=3  VectorParamsAs1DForOutWhenUnconnected=off
  Ldr : Outport  Port=4  VectorParamsAs1DForOutWhenUnconnected=off
  wires:
  Lqs1/1 -> Integrator/1
  Vqs/1 -> Lqs1/1
  W/1 -> Product1/1, Product3/1, W-Wr/1
  Product1/1 -> Lqs1/3
  Lds1/1 -> Integrator1/1
  Vds/1 -> Lds1/1
  Product3/1 -> Lds1/3
  Integrator/1 -> Lqs/1, Product3/2
  Product5/1 -> Lqr1/2
  Lqr1/1 -> Integrator2/1
  Integrator2/1 -> Lqr/1, Product2/1
  Iqs/1 -> Rs/1
  Rs/1 -> Lqs1/2
  Integrator1/1 -> Lds/1, Product1/2
  Rs1/1 -> Lds1/2
  Ids/1 -> Rs1/1
  W-Wr/1 -> Product5/2, Product2/2
  Iqr/1 -> Rr1/1
  Rr1/1 -> Lqr1/1
  Wr/1 -> W-Wr/2
  Ldr1/1 -> Integrator3/1
  Integrator3/1 -> Ldr/1, Product5/1
  Rr2/1 -> Ldr1/1
  Idr/1 -> Rr2/1
  Product2/1 -> Ldr1/2
